simulink model "windtest"  (Simulink 8.3)
settings: Solver=ode5  SolverMode=SingleTasking  StartTime=0.0  StopTime=15  FixedStep=0.01  RelTol=1e-3  AbsTol=1e-6
settings Model: Creator=ikko  LastModifiedBy=ikko
settings DataIOCC: LimitDataPoints=off  SignalLoggingName=logsOut
settings OptimizationCC: BooleanDataType=off  ExpressionDepthLimit=2147483647  InitFltsAndDblsToZero=on
settings DebuggingCC: SaveWithParameterizedLinksMsg=none  CheckExecutionContextPreStartOutputMsg=on  CheckExecutionContextRuntimeOutputMsg=on  SignalResolutionControl=TryResolveAllWithWarning  SolverPrmCheckMsg=none  MultiTaskDSMMsg=warning  MultiTaskCondExecSysMsg=none  FcnCallInpInsideContextMsg=EnableAllAsWarning  StrictBusMsg=None
settings HardwareCC: TargetUnknown=on
settings RTWCC: TemplateMakefile=grt_vc.tmf  IncludeERTFirstTime=on
settings GRTTargetCC: TargetFcnLib=ansi_tfl_tmw.mat

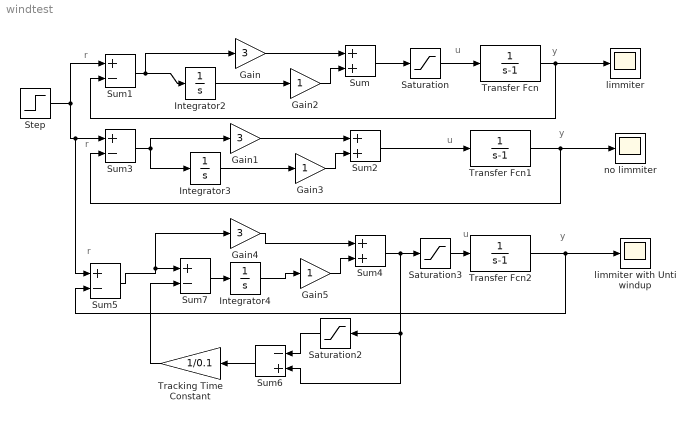
== system windtest ==
  note: r
  note: r
  note: r
  note: u
  note: u
  note: u
  note: y
  note: y
  note: y
  Gain : Gain  Gain=3  SaturateOnIntegerOverflow=on  OutDataTypeStr=Inherit: Same as input  ParamDataTypeStr=Inherit: Same as input
  Gain1 : Gain  Gain=3  SaturateOnIntegerOverflow=on  OutDataTypeStr=Inherit: Same as input  ParamDataTypeStr=Inherit: Same as input
  Gain2 : Gain  SaturateOnIntegerOverflow=on  OutDataTypeStr=Inherit: Same as input  ParamDataTypeStr=Inherit: Same as input
  Gain3 : Gain  SaturateOnIntegerOverflow=on  OutDataTypeStr=Inherit: Same as input  ParamDataTypeStr=Inherit: Same as input
  Gain4 : Gain  Gain=3  SaturateOnIntegerOverflow=on  OutDataTypeStr=Inherit: Same as input  ParamDataTypeStr=Inherit: Same as input
  Gain5 : Gain  SaturateOnIntegerOverflow=on  OutDataTypeStr=Inherit: Same as input  ParamDataTypeStr=Inherit: Same as input
  Integrator2 : Integrator  UpperSaturationLimit=1  LowerSaturationLimit=-1
  Integrator3 : Integrator  UpperSaturationLimit=1  LowerSaturationLimit=-1
  Integrator4 : Integrator  UpperSaturationLimit=1  LowerSaturationLimit=-1
  Saturation : Saturate  UpperLimit=1  LowerLimit=-1
      settings: AttributesFormatString=Upperlimit=%<UpperLimit>\nLowerLimit=%<LowerLimit>
  Saturation2 : Saturate  UpperLimit=1  LowerLimit=-1
      settings: AttributesFormatString=Upperlimit=%<UpperLimit>\nLowerLimit=%<LowerLimit>
  Saturation3 : Saturate  UpperLimit=1  LowerLimit=-1
      settings: AttributesFormatString=Upperlimit=%<UpperLimit>\nLowerLimit=%<LowerLimit>
  Step : Step  After=0.7  SampleTime=0
  Sum : Sum  SaturateOnIntegerOverflow=on  InputSameDT=on  OutDataTypeStr=Inherit: Same as first input
  Sum{1,3,5,7} (4 alike) : Sum  Inputs=+-  SaturateOnIntegerOverflow=on  InputSameDT=on  OutDataTypeStr=Inherit: Same as first input
  Sum2 : Sum  SaturateOnIntegerOverflow=on  InputSameDT=on  OutDataTypeStr=Inherit: Same as first input
  Sum4 : Sum  SaturateOnIntegerOverflow=on  InputSameDT=on  OutDataTypeStr=Inherit: Same as first input
  Sum6 : Sum  Inputs=-+  SaturateOnIntegerOverflow=on  InputSameDT=on  OutDataTypeStr=Inherit: Same as first input
  Tracking Time Constant : Gain  Gain=1/0.1  SaturateOnIntegerOverflow=on  OutDataTypeStr=Inherit: Same as input  ParamDataTypeStr=Inherit: Same as input
  Transfer Fcn : TransferFcn  Denominator=[1 -1]
  Transfer Fcn1 : TransferFcn  Denominator=[1 -1]
  Transfer Fcn2 : TransferFcn  Denominator=[1 -1]
  limmiter : Scope
      settings: TickLabels=on  TimeRange=15  YMin=-3  YMax=3
  limmiter with Unti windup : Scope
      settings: TickLabels=on  TimeRange=15  YMin=-3  YMax=3
  no limmiter : Scope
      settings: TickLabels=on  TimeRange=15  YMin=-3  YMax=3
  wires:
  Gain/1 -> Sum/1
  Saturation/1 -> Transfer Fcn/1
  Gain2/1 -> Sum/2
  Sum/1 -> Saturation/1
  Integrator2/1 -> Gain2/1
  Sum1/1 -> Gain/1, Integrator2/1
  Transfer Fcn/1 -> limmiter/1, Sum1/2
  Gain1/1 -> Sum2/1
  Sum2/1 -> Transfer Fcn1/1
  Gain3/1 -> Sum2/2
  Integrator3/1 -> Gain3/1
  Sum3/1 -> Integrator3/1, Gain1/1
  Transfer Fcn1/1 -> Sum3/2, no limmiter/1
  Step/1 -> Sum1/1, Sum3/1, Sum5/1
  Gain4/1 -> Sum4/1
  Transfer Fcn2/1 -> Sum5/2, limmiter with Unti windup/1
  Saturation2/1 -> Sum6/1
  Saturation3/1 -> Transfer Fcn2/1
  Sum4/1 -> Sum6/2, Saturation2/1, Saturation3/1
  Sum7/1 -> Integrator4/1
  Integrator4/1 -> Gain5/1
  Gain5/1 -> Sum4/2
  Sum5/1 -> Gain4/1, Sum7/1
  Tracking Time Constant/1 -> Sum7/2
  Sum6/1 -> Tracking Time Constant/1
